simulink model "xhand_sphere_tube_r2021b"  (R2021b)
settings: Solver=VariableStepAuto  StartTime=0.0  StopTime=20  RelTol=1e-3
InitFcn:
  | radium=0.045
undefined symbols (not defined in the file): X, Y, Z
libraries: sm_lib x120, nesl_utility x26, Contact_Forces_Lib x21
(part 1 of 4)
settings Model: Creator=hp  LastModifiedBy=majiaji
settings SolverCC: ZeroCrossAlgorithm=Adaptive  AlgebraicLoopSolver=TrustRegion
settings DebuggingCC: RTPrefix=none  StringTruncationChecking=none  AlgebraicLoopMsg=none  ArtificialAlgebraicLoopMsg=none  SaveWithDisabledLinksMsg=none  SaveWithParameterizedLinksMsg=none  SignalResolutionControl=None  MaxConsecutiveZCsMsg=none  MaskedZcDiagnostic=none  IgnoredZcDiagnostic=none  InheritedTsInSrcMsg=none  MultiTaskCondExecSysMsg=none  MultiTaskRateTransMsg=warning  TasksWithSamePriorityMsg=none  SigSpecEnsureSampleTimeMsg=none  IntegerOverflowMsg=none  Int32ToFloatConvMsg=none  ParameterDowncastMsg=none  ParameterOverflowMsg=none  ParameterPrecisionLossMsg=none  ParameterTunabilityLossMsg=none  FcnCallInpInsideContextMsg=warning  UnconnectedInputMsg=none  UnconnectedOutputMsg=none  UnconnectedLineMsg=none  FrameProcessingCompatibilityMsg=none  BusObjectLabelMismatch=none  RootOutportRequireBusObject=none  UnknownTsInhSupMsg=none  ModelReferenceDataLoggingMessage=none  ModelReferenceSymbolNameMessage=none  ModelReferenceExtraNoncontSigs=none  OperatingPointInterfaceChecksumMismatchMsg=none  NonCurrentReleaseOperatingPointMsg=warning  InitInArrayFormatMsg=none  SFMachineParentedDataDiag=warning  IntegerSaturationMsg=none  UnitsInconsistencyMsg=none
settings DiagnosticsConfigSet: SimMechanicsInvalidVisualProperty=none  SimMechanicsCrossSectionNullEdge=none  SimMechanicsUnconnectedFramePorts=none  SimMechanicsUnconnectedGeometryPorts=none  SimMechanicsRedundantBlock=none  SimMechanicsConflictingReferenceFrames=none  SimMechanicsRigidlyBoundBlock=none  SimMechanicsUnsatisfiedHighPriorityTargets=none  SimMechanicsJointTargetOverSpecification=none

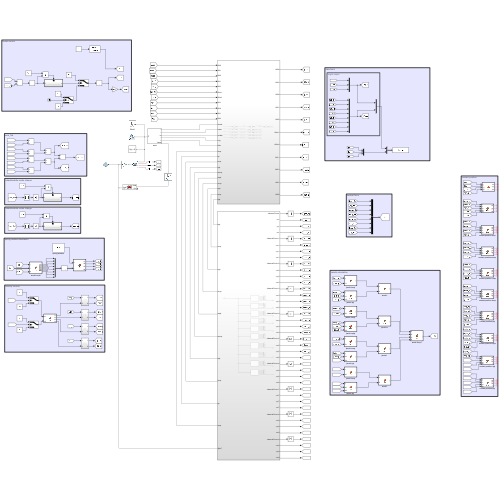
[thumbnail: Simulink's stored preview of the top-level diagram]
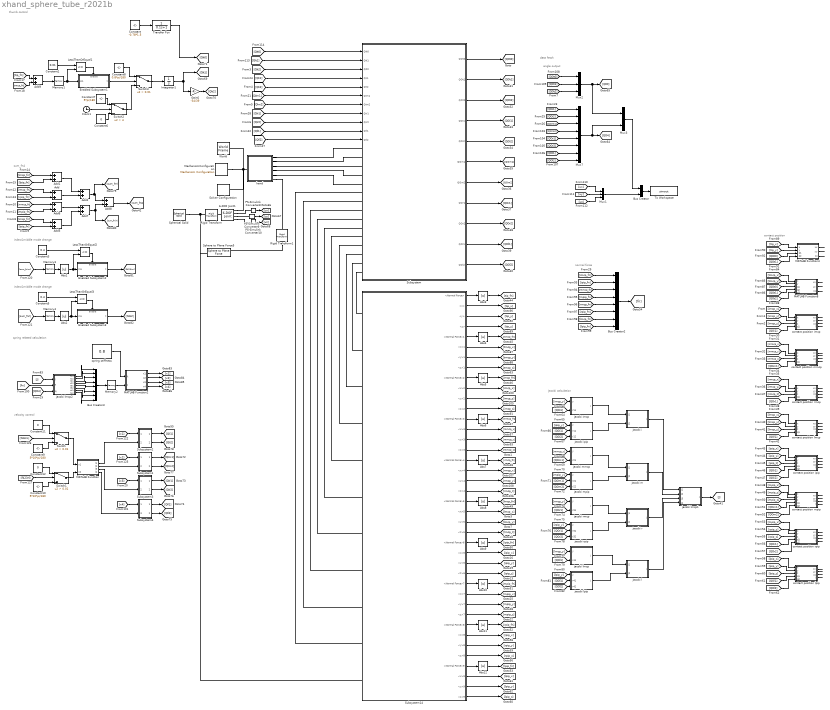
== system xhand_sphere_tube_r2021b ==
  note: spring related calculation
  note: velocity control
  note: thumb control
  note: data fetch
  note: angle output
  note: sum_fn4
  note: contact position
  note: Jacobi calculation
  note: normal force
  note: index&middle mode change
  note: index&middle mode change
  6-DOF Joint1 : sm_lib/Joints/6-DOF Joint  JointMode=Normal  SenseConstraintForce=off  SenseConstraintForceX=off  SenseConstraintForceY=off  SenseConstraintForceZ=off  SenseConstraintTorque=off  SenseConstraintTorqueX=off  SenseConstraintTorqueY=off  SenseConstraintTorqueZ=off  SenseTotalForce=off  SenseTotalForceX=off  SenseTotalForceY=off  SenseTotalForceZ=off  SenseTotalTorque=off  SenseTotalTorqueX=off  SenseTotalTorqueY=off  SenseTotalTorqueZ=off  CompositeWrenchDir=FollowerOnBase  CompositeWrenchFrame=BaseFrame  PxEquilibriumPosition=0  PxEquilibriumPositionUnits=m  PxSpringStiffness=0  PxSpringStiffnessUnits=N/m  PxDampingCoefficient=0  PxDampingCoefficientUnits=N/(m/s)  PxTorqueActuationMode=NoTorque  PxMotionActuationMode=ComputedMotion  PxSensePosition=on  PxSenseVelocity=off  PxSenseAcceleration=off  PxSenseTorqueForce=off  PxSenseLowerLimitTorqueForce=off  PxSenseUpperLimitTorqueForce=off  PxLowerLimitSpecify=off  PxLowerLimitBound=-1  PxLowerLimitBoundUnits=m  PxLowerLimitStiffness=1e6  PxLowerLimitStiffnessUnits=N/m  PxLowerLimitDamping=1e3  PxLowerLimitDampingUnits=N/(m/s)  PxLowerLimitTransitionRegionWidth=1e-4  PxLowerLimitTransitionRegionWidthUnits=m  PxUpperLimitSpecify=off  PxUpperLimitBound=1  PxUpperLimitBoundUnits=m  PxUpperLimitStiffness=1e6  PxUpperLimitStiffnessUnits=N/m  PxUpperLimitDamping=1e3  PxUpperLimitDampingUnits=N/(m/s)  PxUpperLimitTransitionRegionWidth=1e-4  PxUpperLimitTransitionRegionWidthUnits=m  PxPositionTargetSpecify=off  PxPositionTargetPriority=High  PxPositionTargetValue=0  PxPositionTargetValueUnits=m  PxVelocityTargetSpecify=off  PxVelocityTargetPriority=High  PxVelocityTargetValue=0  PxVelocityTargetValueUnits=m/s  PyEquilibriumPosition=0  PyEquilibriumPositionUnits=m  PySpringStiffness=0  PySpringStiffnessUnits=N/m  PyDampingCoefficient=0  PyDampingCoefficientUnits=N/(m/s)  PyTorqueActuationMode=NoTorque  PyMotionActuationMode=ComputedMotion  PySensePosition=on  PySenseVelocity=off  PySenseAcceleration=off  PySenseTorqueForce=off  PySenseLowerLimitTorqueForce=off  PySenseUpperLimitTorqueForce=off  PyLowerLimitSpecify=off  PyLowerLimitBound=-1  PyLowerLimitBoundUnits=m  PyLowerLimitStiffness=1e6  PyLowerLimitStiffnessUnits=N/m  PyLowerLimitDamping=1e3  PyLowerLimitDampingUnits=N/(m/s)  PyLowerLimitTransitionRegionWidth=1e-4  PyLowerLimitTransitionRegionWidthUnits=m  PyUpperLimitSpecify=off  PyUpperLimitBound=1  PyUpperLimitBoundUnits=m  PyUpperLimitStiffness=1e6  PyUpperLimitStiffnessUnits=N/m  PyUpperLimitDamping=1e3  PyUpperLimitDampingUnits=N/(m/s)  PyUpperLimitTransitionRegionWidth=1e-4  PyUpperLimitTransitionRegionWidthUnits=m  PyPositionTargetSpecify=off  PyPositionTargetPriority=High  PyPositionTargetValue=0  PyPositionTargetValueUnits=m  PyVelocityTargetSpecify=off  PyVelocityTargetPriority=High  PyVelocityTargetValue=0  PyVelocityTargetValueUnits=m/s  PzEquilibriumPosition=0  PzEquilibriumPositionUnits=m  PzSpringStiffness=0  PzSpringStiffnessUnits=N/m  PzDampingCoefficient=0  PzDampingCoefficientUnits=N/(m/s)  PzTorqueActuationMode=NoTorque  PzMotionActuationMode=ComputedMotion  PzSensePosition=on  PzSenseVelocity=off  PzSenseAcceleration=off  PzSenseTorqueForce=off  PzSenseLowerLimitTorqueForce=off  PzSenseUpperLimitTorqueForce=off  PzLowerLimitSpecify=off  PzLowerLimitBound=-1  PzLowerLimitBoundUnits=m  PzLowerLimitStiffness=1e6  PzLowerLimitStiffnessUnits=N/m  PzLowerLimitDamping=1e3  PzLowerLimitDampingUnits=N/(m/s)  PzLowerLimitTransitionRegionWidth=1e-4  PzLowerLimitTransitionRegionWidthUnits=m  PzUpperLimitSpecify=off  PzUpperLimitBound=1  PzUpperLimitBoundUnits=m  PzUpperLimitStiffness=1e6  PzUpperLimitStiffnessUnits=N/m  PzUpperLimitDamping=1e3  PzUpperLimitDampingUnits=N/(m/s)  PzUpperLimitTransitionRegionWidth=1e-4  PzUpperLimitTransitionRegionWidthUnits=m  PzPositionTargetSpecify=off  PzPositionTargetPriority=High  PzPositionTargetValue=-0.01  PzPositionTargetValueUnits=m  PzVelocityTargetSpecify=off  PzVelocityTargetPriority=High  PzVelocityTargetValue=0  PzVelocityTargetValueUnits=m/s  SphDefPosRotationMethod=None  SphDefPosRotationAngleUnits=deg  SphDefPosRotationStandardAxis=+Z  SphDefPosRotationAngle=0.0  SphDefPosRotationArbitraryAxis=[0 0 1]  SphDefPosFollAlignAxisA=+X  SphDefPosBaseAlignAxisA=+Y  SphDefPosFollAlignAxisB=+Y  SphDefPosBaseAlignAxisB=+Z  SphDefPosRotationSequenceAxes=FollowerAxes  SphDefPosRotationSequence=XYX  SphDefPosRotationSequenceAngles=[0 0 0]  SphDefPosRotationSequenceAnglesUnits=deg  SphDefPosRotationMatrix=[1 0 0; 0 1 0; 0 0 1]  SphEqPosRotationMethod=None  SphEqPosRotationAngleUnits=deg  SphEqPosRotationStandardAxis=+Z  SphEqPosRotationAngle=0.0  SphEqPosRotationArbitraryAxis=[0 0 1]  SphEqPosFollAlignAxisA=+X  SphEqPosBaseAlignAxisA=+Y  SphEqPosFollAlignAxisB=+Y  SphEqPosBaseAlignAxisB=+Z  SphEqPosRotationSequenceAxes=FollowerAxes  SphEqPosRotationSequence=XYX  SphEqPosRotationSequenceAngles=[0 0 0]  SphEqPosRotationSequenceAnglesUnits=deg  SphEqPosRotationMatrix=[1 0 0; 0 1 0; 0 0 1]  SphSpringStiffness=0  SphSpringStiffnessUnits=N*m/deg  SphDampingCoefficient=0  SphDampingCoefficientUnits=N*m/(deg/s)  SphActuateTorqueX=off  SphActuateTorqueY=off  SphActuateTorqueZ=off  SphActuateTorque=off  SphTorqueActuationMode=NoTorque  SphMotionActuationMode=ComputedMotion  SphActuationFrame=BaseFrame  SphSensePosition=off  SphSenseVelocityX=off  SphSenseVelocityY=off  SphSenseVelocityZ=off  SphSenseVelocity=off  SphSenseAccelerationX=off  SphSenseAccelerationY=off  SphSenseAccelerationZ=off  SphSenseAcceleration=off  SphSenseTorqueX=off  SphSenseTorqueY=off  SphSenseTorqueZ=off  SphSenseTorqueForce=off  SphSenseLowerLimitTorqueMag=off  SphSenseUpperLimitTorqueMag=off  SphSensingFrame=BaseFrame  SphLowerLimitSpecify=off  SphLowerLimitBound=15  SphLowerLimitBoundUnits=deg  SphLowerLimitStiffness=1e4  SphLowerLimitStiffnessUnits=N*m/deg  SphLowerLimitDamping=10  SphLowerLimitDampingUnits=N*m/(deg/s)  SphLowerLimitTransitionRegionWidth=0.1  SphLowerLimitTransitionRegionWidthUnits=deg  SphUpperLimitSpecify=off  SphUpperLimitBound=45  SphUpperLimitBoundUnits=deg  SphUpperLimitStiffness=1e4  SphUpperLimitStiffnessUnits=N*m/deg  SphUpperLimitDamping=10  SphUpperLimitDampingUnits=N*m/(deg/s)  SphUpperLimitTransitionRegionWidth=0.1  SphUpperLimitTransitionRegionWidthUnits=deg  SphPositionTargetRotationMethod=None  SphPositionTargetRotationAngleUnits=deg  SphPositionTargetRotationStandardAxis=+Z  SphPositionTargetRotationAngle=0.0  SphPositionTargetRotationArbitraryAxis=[0 0 1]  SphPositionTargetFollAlignAxisA=+X  SphPositionTargetBaseAlignAxisA=+Y  SphPositionTargetFollAlignAxisB=+Y  SphPositionTargetBaseAlignAxisB=+Z  SphPositionTargetRotationSequenceAxes=FollowerAxes  SphPositionTargetRotationSequence=XYX  SphPositionTargetRotationSequenceAngles=[0 0 0]  SphPositionTargetRotationSequenceAnglesUnits=deg  SphPositionTargetRotationMatrix=[1 0 0; 0 1 0; 0 0 1]  SphPositionTargetSpecify=off  SphPositionTargetPriority=High  SphVelocityTargetValue=[0 0 0]  SphVelocityTargetValueUnits=deg/s  SphVelocityTargetSpecify=off  SphVelocityTargetPriority=High  SphVelocityTargetInFollowerFrame=on
  Abs{1..12} (12 alike) : Abs
  Add{,1..2,5..9} (8 alike) : Sum
  Bus Creator : BusCreator  Inputs=2
  Bus Creator2 : BusCreator  Inputs=8
  Bus Creator3 : BusCreator  Inputs=8
  Clock1 : Clock
  Constant : Constant  Value=-0.78*1.5
  Constant1 : Constant  Value=0.01
  Constant10 : Constant  Value=5*10*pi/180
  Constant11 : Constant  Value=0
  Constant12 : Constant  Value=0
  Constant3 : Constant  Value=0.4
  Constant5 : Constant  Value=0.4
  Constant6 : Constant  Value=0
  Constant7 : Constant  Value=5*pi/180
  Constant8 : Constant  Value=0.8*pi/180
  Constant9 : Constant  Value=5*10*pi/180
  Enabled Subsystem1 : Subsystem  TreatAsAtomicUnit=on
  Enabled Subsystem2 : Subsystem  TreatAsAtomicUnit=on
  Enabled Subsystem3 : Subsystem  TreatAsAtomicUnit=on
  Gain6 : Gain  Gain=-34/39
  Integrator1 : Integrator
  LessThanOrEqual1 : RelationalOperator  Operator=<=  OutDataTypeStr=boolean  RndMeth=Simplest
  LessThanOrEqual2 : RelationalOperator  Operator=<=  OutDataTypeStr=boolean  RndMeth=Simplest
  LessThanOrEqual3 : RelationalOperator  Operator=<=  OutDataTypeStr=boolean  RndMeth=Simplest
  MATLAB Function : MATLAB Function  TreatAsAtomicUnit=on
  MATLAB Function2 : MATLAB Function  TreatAsAtomicUnit=on
  MATLAB Function4 : MATLAB Function  Description=通过球心对平面的投影，得到了接触点的位置。  TreatAsAtomicUnit=on
  MATLAB Function8 : MATLAB Function  Description=通过球心对平面的投影，得到了接触点的位置。  TreatAsAtomicUnit=on
  MechanismConfiguration : sm_lib/Utilities/Mechanism Configuration  UniformGravity=Constant  GravityVector=[0 0 -9.8]  GravityUnits=m/s^2  LinearizationDelta=0.001  JointModeTransitionNonlinearIterations=2
  Memory{1..4} (4 alike) : Memory
  Mux1 : Mux  Inputs=3
  Mux2 : Mux  Inputs=3
  Mux3 : Mux  Inputs=2
  Mux7 : Mux  Inputs=8
  PS-Simulink Converter10 : nesl_utility/PS-Simulink Converter  PhysicalDomain=network_engine_domain  SubClassName=ps_output  LeftPortType=input  RightPortType=output  PseudoPeriodic=off  Frequencies=[]  Unit=inherit  AffineConversion=off
      settings: SourceProductBaseCode=PW,SS
  PS-Simulink Converter8 : nesl_utility/PS-Simulink Converter  PhysicalDomain=network_engine_domain  SubClassName=ps_output  LeftPortType=input  RightPortType=output  PseudoPeriodic=off  Frequencies=[]  Unit=inherit  AffineConversion=off
      settings: SourceProductBaseCode=PW,SS
  PS-Simulink Converter9 : nesl_utility/PS-Simulink Converter  PhysicalDomain=network_engine_domain  SubClassName=ps_output  LeftPortType=input  RightPortType=output  PseudoPeriodic=off  Frequencies=[]  Unit=inherit  AffineConversion=off
      settings: SourceProductBaseCode=PW,SS
  Rigid Transform : sm_lib/Frames and Transforms/Rigid Transform  TranslationMethod=Cartesian  TranslationStandardOffset=0  TranslationLengthUnit=mm  TranslationStandardAxis=+Z  TranslationCartesianOffset=[-6 -12 -1000*radium]  TranslationROffset=0  TranslationROffsetUnits=m  TranslationZOffset=0  TranslationZOffsetUnits=m  TranslationThetaOffset=0  TranslationThetaOffsetUnits=deg  RotationMethod=None  RotationAngleUnits=deg  RotationStandardAxis=+Z  RotationAngle=0.0  RotationArbitraryAxis=[0 0 1]  FollAlignAxisA=+X  BaseAlignAxisA=+Y  FollAlignAxisB=+Y  BaseAlignAxisB=+Z  RotationSequenceAxes=FollowerAxes  RotationSequence=XYX  RotationSequenceAngles=[0 0 0]  RotationSequenceAnglesUnits=deg  RotationMatrix=[1 0 0; 0 1 0; 0 0 1]
  Rigid Transform1 : sm_lib/Frames and Transforms/Rigid Transform  TranslationMethod=Cartesian  TranslationStandardOffset=0  TranslationLengthUnit=mm  TranslationStandardAxis=+Z  TranslationCartesianOffset=[0 0 -4]  TranslationROffset=0  TranslationROffsetUnits=m  TranslationZOffset=0  TranslationZOffsetUnits=m  TranslationThetaOffset=0  TranslationThetaOffsetUnits=deg  RotationMethod=None  RotationAngleUnits=deg  RotationStandardAxis=+Z  RotationAngle=0.0  RotationArbitraryAxis=[0 0 1]  FollAlignAxisA=+X  BaseAlignAxisA=+Y  FollAlignAxisB=+Y  BaseAlignAxisB=+Z  RotationSequenceAxes=FollowerAxes  RotationSequence=XYX  RotationSequenceAngles=[0 0 0]  RotationSequenceAnglesUnits=deg  RotationMatrix=[1 0 0; 0 1 0; 0 0 1]
  Solver Configuration : nesl_utility/Solver Configuration  PhysicalDomain=network_engine_domain  SubClassName=solver  LeftPortType=input  RightPortType=generic  Tones=[]  Harmonics=[]  SimulateNoise=off  Profile=off  UseLocalSampling=off  EnableSwitchedLinearOptims=on  FrequencyDomain=off  UseCCode=off  RelTol=0.001  AbsTol=1e-06  MinStep=1e-09  ToWorkspace=off  RevertToSquareIcSolve=off  NumHomotopyIterations=100  PhasorMode=off  PhasorModeNumHarmonics=1  DoDC=off  ResidualTolerance=1e-09  UseLocalSolver=off  LocalSolverChoice=NE_BACKWARD_EULER_ADVANCER  LocalSolverSampleTime=0.001  DoFixedCost=off  MaxNonlinIter=3  MaxModeIter=2  ComputeImpulses=off  ImpulseIterations=2  LinearAlgebra=auto  EquationFormulation=NE_TIME_EF  DelaysMemoryBudget=1024  AutomaticFiltering=on  FilteringTimeConstant=0.001  PartitionStorageMethod=AS_NEEDED  PartitionMemoryBudget=1024  PartitionMethod=ROBUST
      settings: SourceProductBaseCode=PW,SS
  Sphere to Plane Force5 : Contact_Forces_Lib/3D/Sphere to Plane Force  sphere_rad=radium+0.001  plane_lenx=0.1  plane_leny=0.1  plane_depth=0.01/2*0.5*0.4  force_law=Linear  k_contact=10000  b_contact=1000  pen_full_damp_F=1e-4  pen_exponent=1  custom_param_1=1  custom_param_2=1  friction_law=Stick-Slip Continuous  mu_kinetic=0.7  mu_static=0.9  v_thr=0.5  vis_on=off  vis_opc_en=0  vis_len_plaBz=0.0001  vis_clr=[0.9 0.2 0.2]  vis_opc=0.7
  Spherical Solid : sm_lib/Body Elements/Spherical Solid  GraphicAmbientColor=[0.15 0.15 0.15 1.0]  BasedOnType=Density  CenterOfMass=[0 0 0]  CenterOfMassUnits=m  GraphicDiffuseColor=[0.5 0.5 0.5]  Density=1000  DensityUnits=kg/m^3  DoExposeReferenceFrame=on  GraphicEmissiveColor=[0.0 0.0 0.0 1.0]  ExportEntireGeometry=off  SerializedExposedGeometries=<ExposedGeometries/>  SerializedFrames=<Frames/>  MarkerShape=Sphere  MarkerSize=10  GraphicType=FromGeometry  InertiaType=CalculateFromGeometry  Mass=1  MassUnits=kg  MomentsOfInertia=[1 1 1]  MomentsOfInertiaUnits=kg*m^2  GraphicOpacity=1.0  ProductsOfInertia=[0 0 0]  ProductsOfInertiaUnits=kg*m^2  GraphicShininess=75  GraphicSpecularColor=[0.5 0.5 0.5 1.0]  SphereRadius=radium  SphereRadiusUnits=m  GraphicVisPropType=SimpleVisualProperties
  Subsystem : Subsystem
  Subsystem1 : Subsystem
  Subsystem14 : Subsystem
  Subsystem2 : Subsystem
  Subsystem3 : Subsystem
  Subsystem4 : Subsystem
  Switch : Switch  Criteria=u2 > Threshold  Threshold=0.01
  Switch1 : Switch  Criteria=u2 > Threshold  Threshold=0.01
  Switch2 : Switch  Criteria=u2 > Threshold  Threshold=4
  Switch3 : Switch  Criteria=u2 > Threshold  Threshold=0.01
  To Workspace : ToWorkspace  VariableName=simout  SaveFormat=Timeseries  SampleTime=-1
  Transfer Fcn : TransferFcn  Denominator=[0.1 1]
  World : sm_lib/Frames and Transforms/World Frame
  "contact position imcp " : MATLAB Function  Description=通过球心对平面的投影，得到了接触点的位置。  TreatAsAtomicUnit=on
  contact position ipip : MATLAB Function  Description=通过球心对平面的投影，得到了接触点的位置。  TreatAsAtomicUnit=on
  contact position lmcp : MATLAB Function  Description=通过球心对平面的投影，得到了接触点的位置。  TreatAsAtomicUnit=on
  contact position lpip : MATLAB Function  Description=通过球心对平面的投影，得到了接触点的位置。  TreatAsAtomicUnit=on
  contact position mmcp : MATLAB Function  Description=通过球心对平面的投影，得到了接触点的位置。  TreatAsAtomicUnit=on
  contact position mpip : MATLAB Function  Description=通过球心对平面的投影，得到了接触点的位置。  TreatAsAtomicUnit=on
  contact position rmcp : MATLAB Function  Description=通过球心对平面的投影，得到了接触点的位置。  TreatAsAtomicUnit=on
  contact position rpip : MATLAB Function  Description=通过球心对平面的投影，得到了接触点的位置。  TreatAsAtomicUnit=on
  hand : Subsystem
  jacobi i : MATLAB Function  Description=通过球心对平面的投影，得到了接触点的位置。  TreatAsAtomicUnit=on
  jacobi imcp : MATLAB Function  Description=通过球心对平面的投影，得到了接触点的位置。  TreatAsAtomicUnit=on
  jacobi ipip : MATLAB Function  Description=通过球心对平面的投影，得到了接触点的位置。  TreatAsAtomicUnit=on
  jacobi l : MATLAB Function  Description=通过球心对平面的投影，得到了接触点的位置。  TreatAsAtomicUnit=on
  jacobi lmcp : MATLAB Function  Description=通过球心对平面的投影，得到了接触点的位置。  TreatAsAtomicUnit=on
  jacobi lmcp1 : MATLAB Function  Description=通过球心对平面的投影，得到了接触点的位置。  TreatAsAtomicUnit=on
  jacobi lmcp2 : MATLAB Function  Description=通过球心对平面的投影，得到了接触点的位置。  TreatAsAtomicUnit=on
  jacobi lpip : MATLAB Function  Description=通过球心对平面的投影，得到了接触点的位置。  TreatAsAtomicUnit=on
  jacobi m : MATLAB Function  Description=通过球心对平面的投影，得到了接触点的位置。  TreatAsAtomicUnit=on
  jacobi mmcp : MATLAB Function  Description=通过球心对平面的投影，得到了接触点的位置。  TreatAsAtomicUnit=on
  jacobi mpip : MATLAB Function  Description=通过球心对平面的投影，得到了接触点的位置。  TreatAsAtomicUnit=on
  jacobi r : MATLAB Function  Description=通过球心对平面的投影，得到了接触点的位置。  TreatAsAtomicUnit=on
  jacobi rmcp : MATLAB Function  Description=通过球心对平面的投影，得到了接触点的位置。  TreatAsAtomicUnit=on
  jacobi rpip : MATLAB Function  Description=通过球心对平面的投影，得到了接触点的位置。  TreatAsAtomicUnit=on
  spring stiffness : Constant  Value=0.8
  wires:
  PS-Simulink Converter8/1 -> [ux]
  PS-Simulink Converter9/1 -> [uy]
  PS-Simulink Converter10/1 -> [uz]
  [QIt0] -> Subsystem/1(QIt0)
  [QIt1] -> Subsystem/2(QIt1)
  [QIt2] -> Subsystem/3(QIt2)
  [QIi2] -> Subsystem/5(QIi2)
  [QIi1] -> Subsystem/4(QIi1)
  [QIm2] -> Subsystem/7(QIm2)
  [QIm1] -> Subsystem/6(QIm1)
  [QIr2] -> Subsystem/9(QIr2)
  [QIl2] -> Subsystem/11(QIl2)
  [QIr1] -> Subsystem/8(QIr1)
  [QIl1] -> Subsystem/10(QIl1)
  Subsystem/3(QOt2) -> [QOt2]
  Subsystem/1(QOt0) -> [QOt0]
  Subsystem/2(QOt1) -> [QOt1]
  Subsystem/5(QOi2) -> [QOi2]
  Subsystem/4(QOi1) -> [QOi1]
  Subsystem/7(QOm2) -> [QOm2]
  Subsystem/6(QOm1) -> [QOm1]
  Subsystem/9(QOr2) -> [QOr2]
  Subsystem/11(QOl2) -> [QOl2]
  Subsystem/8(QOr1) -> [QOr1]
  Subsystem/10(QOl1) -> [QOl1]
  [ux] -> Mux1/1
  [QOm1] -> Mux7/3
  [QOi2] -> Mux7/2
  [QOm2] -> Mux7/4
  Mux3/1 -> Bus Creator/1
  Mux1/1 -> Bus Creator/2
  [QOt0] -> Mux2/1
  [QOl1] -> Mux7/7
  [uy] -> Mux1/2
  [QOr2] -> Mux7/6
  [QOi1] -> Mux7/1
  [QOt1] -> Mux2/2
  [uz] -> Mux1/3
  [QOl2] -> Mux7/8
  Mux2/1 -> Mux3/1, [QOt]
  [QOr1] -> Mux7/5
  Bus Creator/1 -> To Workspace/1
  [QOt2] -> Mux2/3
  Mux7/1 -> Mux3/2, [QO4]
  Add/1 -> Add2/2
  [rmcp_fn] -> Add/1
  [mmcp_fn] -> Add6/1
  [lpip_fn] -> Add1/2
  [rpip_fn] -> Add/2
  Add2/1 -> [sum_fnrl], Add8/1
  Add8/1 -> [sum_fn4]
  [ipip_fn] -> Add5/2
  [lmcp_fn] -> Add1/1
  [imcp_fn] -> Add5/1
  Add6/1 -> Add7/1
  [mpip_fn] -> Add6/2
  Add1/1 -> Add2/1
  Add5/1 -> Add7/2
  Add7/1 -> Add8/2, [sum_fnim]
  Constant7/1 -> Switch2/1
  Switch2/1 -> Switch3/3
  Clock1/1 -> Switch2/2
  Constant6/1 -> Switch2/3
  Gain6/1 -> [QIt2]
  Enabled Subsystem1/1(t) -> Switch3/2
  LessThanOrEqual1/1 -> Enabled Subsystem1/Enable
  Memory1/1 -> Enabled Subsystem1/1(In1), LessThanOrEqual1/2
  Constant1/1 -> LessThanOrEqual1/1
  Add9/1 -> Memory1/1
  Integrator1/1 -> Gain6/1, [QIt1]
  Constant8/1 -> Switch3/1
  Transfer Fcn/1 -> [QIt0]
  Switch3/1 -> Integrator1/1
  [tmcp_fn] -> Add9/2
  [tip_fn] -> Add9/1
  Constant/1 -> Transfer Fcn/1
  Subsystem14/1(<Normal Force>) -> Abs3/1
  Subsystem14/2(<x>) -> [tip_x]
  Subsystem14/3(<y>) -> [tip_y]
  Subsystem14/4(<z>) -> [tip_z]
  Subsystem14/5(<Normal Force>1) -> Abs4/1
  Subsystem14/6(<x>1) -> [tmcp_x]
  Subsystem14/7(<y>1) -> [tmcp_y]
  Subsystem14/8(<z>1) -> [tmcp_z]
  Subsystem14/9(<Normal Force>2) -> Abs5/1
  Subsystem14/10(<x>2) -> [imcp_x]
  Subsystem14/11(<y>2) -> [imcp_y]
  Subsystem14/12(<z>2) -> [imcp_z]
  Subsystem14/13(<Normal Force>3) -> Abs6/1
  Subsystem14/14(<x>3) -> [mmcp_x]
  Subsystem14/15(<y>3) -> [mmcp_y]
  Subsystem14/16(<z>3) -> [mmcp_z]
  Subsystem14/17(<Normal Force>4) -> Abs7/1
  Subsystem14/18(<x>4) -> [rmcp_x]
  Subsystem14/19(<y>4) -> [rmcp_y]
  Subsystem14/20(<z>4) -> [rmcp_z]
  Subsystem14/21(<Normal Force>5) -> Abs8/1
  Subsystem14/22(<x>5) -> [lmcp_x]
  Subsystem14/23(<y>5) -> [lmcp_y]
  Subsystem14/24(<z>5) -> [lmcp_z]
  Subsystem14/25(<Normal Force>6) -> Abs9/1
  Subsystem14/26(<x>6) -> [ipip_x]
  Subsystem14/27(<y>6) -> [ipip_y]
  Subsystem14/28(<z>6) -> [ipip_z]
  Subsystem14/29(<Normal Force>7) -> Abs10/1
  Subsystem14/30(<x>7) -> [mpip_x]
  Subsystem14/31(<y>7) -> [mpip_y]
  Subsystem14/32(<z>7) -> [mpip_z]
  Subsystem14/33(<Normal Force>8) -> Abs11/1
  Subsystem14/34(<x>8) -> [rpip_x]
  Subsystem14/35(<y>8) -> [rpip_y]
  Subsystem14/36(<z>8) -> [rpip_z]
  Subsystem14/37(<Normal Force>9) -> Abs12/1
  Subsystem14/38(<x>9) -> [lpip_x]
  Subsystem14/39(<y>9) -> [lpip_y]
  Subsystem14/40(<z>9) -> [lpip_z]
  [QOi1] -> contact position ipip/4(q1)
  [rmcp_x] -> contact position rmcp/1(x)
  [QOt1] -> MATLAB Function4/4(q2)
  [mmcp_x] -> contact position mmcp/1(x)
  [rpip_y] -> contact position rpip/2(y)
  [mmcp_z] -> contact position mmcp/3(z)
  [QOt1] -> MATLAB Function8/4(q2)
  [QOi2] -> contact position ipip/5(q2)
  [mpip_x] -> contact position rpip/1(x)
  [rmcp_y] -> contact position rmcp/2(y)
  [imcp_z] -> "contact position imcp "/3(z)
  [lmcp_z] -> contact position lmcp/3(z)
  [mpip_x] -> contact position mpip/1(x)
  [mpip_y] -> contact position mpip/2(y)
  [lpip_x] -> contact position lpip/1(x)
  [tmcp_y] -> MATLAB Function8/2(y)
  [rpip_z] -> contact position rpip/3(z)
  [QOi1] -> "contact position imcp "/4(q1)
  [lpip_z] -> contact position lpip/3(z)
  [ipip_z] -> contact position ipip/3(z)
  [mpip_z] -> contact position mpip/3(z)
  [tmcp_x] -> MATLAB Function8/1(x)
  [QOl1] -> contact position lmcp/4(q1)
  [QOr2] -> contact position rpip/5(q2)
  [lmcp_x] -> contact position lmcp/1(x)
  [ipip_y] -> contact position ipip/2(y)
  [QOt2] -> MATLAB Function8/5(q3)
  [QOl1] -> contact position lpip/4(q1)
  [QOm1] -> contact position mpip/4(q1)
  [mmcp_y] -> contact position mmcp/2(y)
  [tip_x] -> MATLAB Function4/1(x)
  [lpip_y] -> contact position lpip/2(y)
  [QOm1] -> contact position mmcp/4(q1)
  "contact position imcp "/3(zz) -> ?
  contact position mmcp/2(yy) -> ?
  contact position rpip/1(xx) -> ?
  [lmcp_y] -> contact position lmcp/2(y)
  "contact position imcp "/2(yy) -> ?
  contact position lmcp/1(xx) -> ?
  [QOt0] -> MATLAB Function4/3(q1)
  MATLAB Function4/3(zz) -> ?
  contact position mmcp/1(xx) -> ?
  contact position lpip/4(l) -> ?
  contact position lpip/1(xx) -> ?
  [imcp_y] -> "contact position imcp "/2(y)
  contact position lmcp/2(yy) -> ?
  MATLAB Function4/1(xx) -> ?
  [QOl2] -> contact position lpip/5(q2)
  contact position rmcp/4(l) -> ?
  contact position lpip/2(yy) -> ?
  contact position mmcp/3(zz) -> ?
  contact position mpip/3(zz) -> ?
  [QOr1] -> contact position rpip/4(q1)
  [QOt0] -> MATLAB Function8/3(q1)
  contact position rmcp/2(yy) -> ?
  [imcp_x] -> "contact position imcp "/1(x)
  [QOr1] -> contact position rmcp/4(q1)
  contact position mpip/1(xx) -> ?
  contact position lpip/3(zz) -> ?
  contact position ipip/3(zz) -> ?
  [ipip_x] -> contact position ipip/1(x)
  contact position ipip/1(xx) -> ?
  MATLAB Function8/3(zz) -> ?
  contact position rmcp/1(xx) -> ?
  contact position mpip/2(yy) -> ?
  MATLAB Function4/2(yy) -> ?
  contact position rpip/3(zz) -> ?
  contact position lmcp/3(zz) -> ?
  "contact position imcp "/1(xx) -> ?
  MATLAB Function8/1(xx) -> ?
  MATLAB Function8/2(yy) -> ?
  contact position lmcp/4(l) -> ?
  contact position ipip/2(yy) -> ?
  contact position rmcp/3(zz) -> ?
  contact position mpip/4(l) -> ?
  [rmcp_z] -> contact position rmcp/3(z)
  [QOm2] -> contact position mpip/5(q2)
  "contact position imcp "/4(l) -> ?
  [tip_y] -> MATLAB Function4/2(y)
  contact position ipip/4(l) -> ?
  contact position mmcp/4(l) -> ?
  contact position rpip/2(yy) -> ?
  contact position rpip/4(l) -> ?
  [lpip_y] -> jacobi lpip/1(y)
  [ipip_y] -> jacobi ipip/1(y)
  [QOl1] -> jacobi lpip/2(r41)
  jacobi r/1(j) -> jacobi lmcp1/3(j3)
  [mpip_y] -> jacobi mpip/1(y)
  jacobi mmcp/1(j) -> jacobi m/1(j1)
  [QOr1] -> jacobi rmcp/2(r31)
  jacobi lmcp1/1(j) -> [j]
  [QOm2] -> jacobi mpip/3(r22)
  [rpip_y] -> jacobi rpip/1(y)
  jacobi i/1(j) -> jacobi lmcp1/1(j1)
  jacobi lpip/1(j) -> jacobi l/2(j2)
  [mmcp_y] -> jacobi mmcp/1(y)
  [QOi2] -> jacobi ipip/3(r12)
  jacobi l/1(j) -> jacobi lmcp1/4(j4)
  jacobi mpip/1(j) -> jacobi m/2(j2)
  [QOi1] -> jacobi ipip/2(r11)
  [QOl1] -> jacobi lmcp/2(r41)
  jacobi rmcp/1(j) -> jacobi r/1(j1)
  jacobi lmcp/1(j) -> jacobi l/1(j1)
  jacobi rpip/1(j) -> jacobi r/2(j2)
  [lmcp_y] -> jacobi lmcp/1(y)
  jacobi m/1(j) -> jacobi lmcp1/2(j2)
  jacobi ipip/1(j) -> jacobi i/2(j2)
  [QOl2] -> jacobi lpip/3(r42)
  [QOr2] -> jacobi rpip/3(r32)
  [QOr1] -> jacobi rpip/2(r31)
  [QOi1] -> jacobi imcp/2(r11)
  [QOm1] -> jacobi mpip/2(r21)
  [rmcp_y] -> jacobi rmcp/1(y)
  jacobi imcp/1(j) -> jacobi i/1(j1)
  [QOm1] -> jacobi mmcp/2(r21)
  [imcp_y] -> jacobi imcp/1(y)
  [imcp_fn] -> Bus Creator2/1
  [rmcp_fn] -> Bus Creator2/5
  [ipip_fn] -> Bus Creator2/2
  [rpip_fn] -> Bus Creator2/6
  [mmcp_fn] -> Bus Creator2/3
  [lpip_fn] -> Bus Creator2/8
  [lmcp_fn] -> Bus Creator2/7
  [mpip_fn] -> Bus Creator2/4
  Bus Creator2/1 -> [fn]
  Abs3/1 -> [tip_fn]
  Abs4/1 -> [tmcp_fn]
  Abs5/1 -> [imcp_fn]
  Abs6/1 -> [mmcp_fn]
  Abs7/1 -> [rmcp_fn]
  Abs8/1 -> [lmcp_fn]
  Abs9/1 -> [ipip_fn]
  Abs10/1 -> [mpip_fn]
  Abs11/1 -> [rpip_fn]
  Abs12/1 -> [lpip_fn]
  Subsystem3/2(Out2) -> [QIr2]
  [x2] -> Subsystem1/1(In2)
  [x4] -> Subsystem4/1(In2)
  Subsystem2/1(Out1) -> [QIi1]
  MATLAB Function/3(l3) -> Subsystem3/2(2)
  [f423im] -> Switch/2
  MATLAB Function/2(l2) -> Subsystem1/2(In1)
  [x1] -> Subsystem2/1(In1)
  Subsystem4/2(Out2) -> [QIl2]
  Switch1/1 -> MATLAB Function/2(x2)
  MATLAB Function/4(l4) -> Subsystem4/2(3)
  Subsystem1/1(Out1) -> [QIm1]
  Switch/1 -> MATLAB Function/1(x1)
  Subsystem1/2(Out2) -> [QIm2]
  [x3] -> Subsystem3/1(In2)
  Constant12/1 -> Switch1/1
  Constant10/1 -> Switch1/3
  Subsystem3/1(Out1) -> [QIr1]
  Constant9/1 -> Switch/3
  Constant11/1 -> Switch/1
  MATLAB Function/1(l1) -> Subsystem2/2(In2)
  [f423rl] -> Switch1/2
  Subsystem2/2(Out2) -> [QIi2]
  Subsystem4/1(Out1) -> [QIl1]
  [j] -> jacobi lmcp2/1(j)
  MATLAB Function2/1(x1) -> [x1]
  jacobi lmcp2/6(t32) -> Bus Creator3/6
  [fn] -> jacobi lmcp2/2(f)
  MATLAB Function2/3(x3) -> [x3]
  jacobi lmcp2/4(t22) -> Bus Creator3/4
  jacobi lmcp2/7(t41) -> Bus Creator3/7
  jacobi lmcp2/2(t12) -> Bus Creator3/2
  MATLAB Function2/4(x4) -> [x4]
  jacobi lmcp2/1(t11) -> Bus Creator3/1
  Bus Creator3/1 -> Memory2/1
  jacobi lmcp2/8(t42) -> Bus Creator3/8
  [QO4] -> jacobi lmcp2/3(q)
  spring stiffness/1 -> MATLAB Function2/1(k)
  Memory2/1 -> MATLAB Function2/2(t)
  jacobi lmcp2/3(t21) -> Bus Creator3/3
  MATLAB Function2/2(x2) -> [x2]
  jacobi lmcp2/5(t31) -> Bus Creator3/5
  Abs1/1 -> Enabled Subsystem2/1(In1), LessThanOrEqual2/2
  LessThanOrEqual2/1 -> Enabled Subsystem2/Enable
  [sum_fnim] -> Memory3/1
  Enabled Subsystem3/1(t) -> [f423rl]
  Constant3/1 -> LessThanOrEqual2/1
  Constant5/1 -> LessThanOrEqual3/1
  Memory3/1 -> Abs1/1
  Memory4/1 -> Abs2/1
  Enabled Subsystem2/1(t) -> [f423im]
  LessThanOrEqual3/1 -> Enabled Subsystem3/Enable
  [sum_fnrl] -> Memory4/1
  Abs2/1 -> Enabled Subsystem3/1(In1), LessThanOrEqual3/2
  connections:
  Rigid Transform/RConn1 -- 6-DOF Joint1/LConn1
  hand/RConn6 -- Rigid Transform1/LConn1
  MechanismConfiguration/RConn1 -- 6-DOF Joint1/RConn1 -- Solver Configuration/RConn1 -- World/RConn1 -- hand/LConn1
  6-DOF Joint1/RConn2 -- PS-Simulink Converter8/LConn1
  6-DOF Joint1/RConn3 -- PS-Simulink Converter9/LConn1
  6-DOF Joint1/RConn4 -- PS-Simulink Converter10/LConn1
  Rigid Transform1/RConn1 -- Sphere to Plane Force5/RConn1
  hand/RConn1 -- Subsystem/LConn1
  hand/RConn2 -- Subsystem/LConn2
  hand/RConn3 -- Subsystem/LConn3
  hand/RConn4 -- Subsystem/LConn4
  hand/RConn5 -- Subsystem/LConn5
  Spherical Solid/RConn1 -- Sphere to Plane Force5/LConn1 -- Subsystem14/LConn11 -- Rigid Transform/LConn1
  Subsystem14/LConn10 -- Subsystem/LConn6
  Subsystem14/LConn9 -- Subsystem/LConn7
  Subsystem14/LConn8 -- Subsystem/LConn8
  Subsystem14/LConn7 -- Subsystem/LConn9
  Subsystem14/LConn6 -- Subsystem/LConn10
  Subsystem14/LConn5 -- Subsystem/LConn11
  Subsystem14/LConn4 -- Subsystem/LConn12
  Subsystem/LConn13 -- Subsystem14/LConn3
  Subsystem14/LConn2 -- Subsystem/LConn14
  Subsystem14/LConn1 -- Subsystem/LConn15

== system xhand_sphere_tube_r2021b/Enabled Subsystem1 ==
  In1 : Inport
  Enable : EnablePort  PropagateVarSize=During execution
  t : Outport
  wires:
  In1/1 -> t/1

== system xhand_sphere_tube_r2021b/Enabled Subsystem2 ==
  In1 : Inport
  Enable : EnablePort  PropagateVarSize=During execution
  t : Outport
  wires:
  In1/1 -> t/1

== system xhand_sphere_tube_r2021b/Enabled Subsystem3 ==
  In1 : Inport
  Enable : EnablePort  PropagateVarSize=During execution
  t : Outport
  wires:
  In1/1 -> t/1
